simulink model "MHILSimTDFixpoint"  (R2021b)
settings: Solver=VariableStepAuto  StartTime=0.0  StopTime=10.0  RelTol=1e-3
values from neighbouring files (symbols this model uses):
  m = tddbl_model    [HILSimModel.m]
libraries: simulink x54
(part 1 of 2)
settings Model: Creator=berndorfer  LastModifiedBy=berndorfer

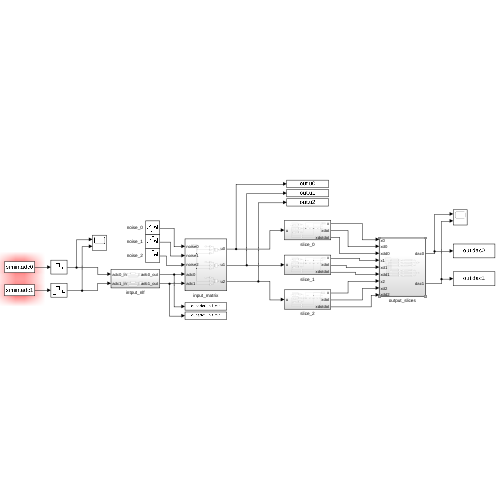
[thumbnail: Simulink's stored preview of the top-level diagram]
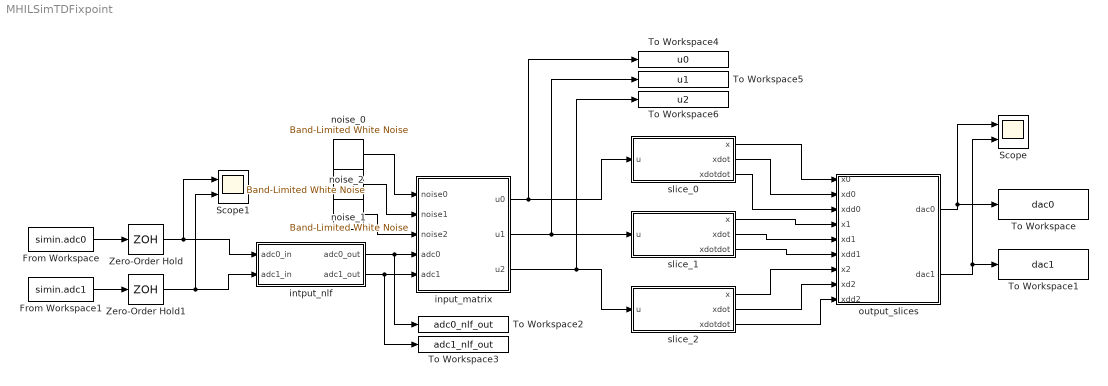
== system MHILSimTDFixpoint ==
  From Workspace : FromWorkspace  VariableName=simin.adc0
  From Workspace1 : FromWorkspace  VariableName=simin.adc1
  Scope : Scope  NumInputPorts=2
  Scope1 : Scope  NumInputPorts=2
  To Workspace : ToWorkspace  VariableName=dac0  SaveFormat=Timeseries  SampleTime=-1
  To Workspace1 : ToWorkspace  VariableName=dac1  SaveFormat=Timeseries  SampleTime=-1
  To Workspace2 : ToWorkspace  VariableName=adc0_nlf_out  SaveFormat=Timeseries  SampleTime=-1
  To Workspace3 : ToWorkspace  VariableName=adc1_nlf_out  SaveFormat=Timeseries  SampleTime=-1
  To Workspace4 : ToWorkspace  VariableName=u0  SaveFormat=Timeseries  SampleTime=-1
  To Workspace5 : ToWorkspace  VariableName=u1  SaveFormat=Timeseries  SampleTime=-1
  To Workspace6 : ToWorkspace  VariableName=u2  SaveFormat=Timeseries  SampleTime=-1
  Zero-Order Hold : ZeroOrderHold  SampleTime=m.t_s
  Zero-Order Hold1 : ZeroOrderHold  SampleTime=m.t_s
  input_matrix : Subsystem
  intput_nlf : Subsystem
  noise_0 : simulink/Sources/Band-Limited White Noise  Cov=[m.n0_power*m.t_s]  Ts=m.t_s  seed=[23341]
  noise_1 : simulink/Sources/Band-Limited White Noise  Cov=[m.n1_power*m.t_s]  Ts=m.t_s  seed=[23341]
  noise_2 : simulink/Sources/Band-Limited White Noise  Cov=[m.n2_power*m.t_s]  Ts=m.t_s  seed=[23341]
  output_slices : Subsystem
  slice_0 : Subsystem
  slice_1 : Subsystem
  slice_2 : Subsystem
  wires:
  slice_1/1(x) -> output_slices/4(x1)
  slice_1/2(xdot) -> output_slices/5(xd1)
  slice_0/2(xdot) -> output_slices/2(xd0)
  slice_0/1(x) -> output_slices/1(x0)
  slice_2/1(x) -> output_slices/7(x2)
  slice_2/2(xdot) -> output_slices/8(xd2)
  input_matrix/2(u1) -> To Workspace5/1, slice_1/1(u)
  input_matrix/1(u0) -> To Workspace4/1, slice_0/1(u)
  input_matrix/3(u2) -> To Workspace6/1, slice_2/1(u)
  intput_nlf/1(adc0_out) -> To Workspace2/1, input_matrix/4(adc0)
  intput_nlf/2(adc1_out) -> To Workspace3/1, input_matrix/5(adc1)
  output_slices/2(dac1) -> Scope/2, To Workspace1/1
  output_slices/1(dac0) -> Scope/1, To Workspace/1
  noise_0/1 -> input_matrix/1(noise0)
  noise_1/1 -> input_matrix/2(noise1)
  noise_2/1 -> input_matrix/3(noise2)
  From Workspace/1 -> Zero-Order Hold/1
  From Workspace1/1 -> Zero-Order Hold1/1
  Zero-Order Hold1/1 -> Scope1/2, intput_nlf/2(adc1_in)
  Zero-Order Hold/1 -> intput_nlf/1(adc0_in), Scope1/1
  slice_0/3(xdotdot) -> output_slices/3(xdd0)
  slice_1/3(xdotdot) -> output_slices/6(xdd1)
  slice_2/3(xdotdot) -> output_slices/9(xdd2)

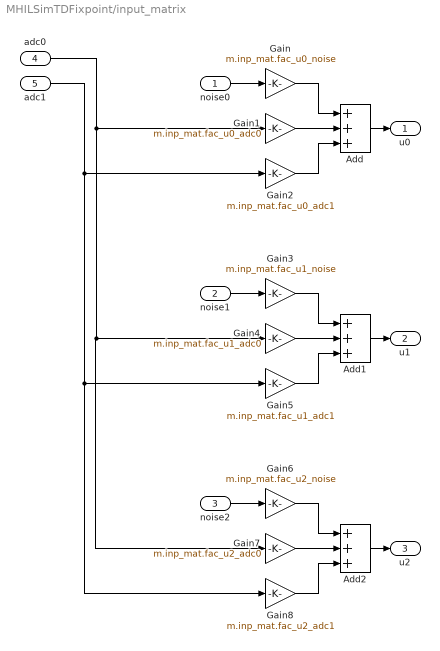
== system MHILSimTDFixpoint/input_matrix ==
  noise0 : Inport
  noise1 : Inport  Port=2
  noise2 : Inport  Port=3
  adc0 : Inport  Port=4
  adc1 : Inport  Port=5
  Add : Sum  Inputs=+++  OutDataTypeStr=m.datatype.slice
  Add1 : Sum  Inputs=+++  OutDataTypeStr=m.datatype.slice
  Add2 : Sum  Inputs=+++  OutDataTypeStr=m.datatype.slice
  Gain : Gain  Gain=m.inp_mat.fac_u0_noise  OutDataTypeStr=m.datatype.slice
  Gain1 : Gain  Gain=m.inp_mat.fac_u0_adc0  OutDataTypeStr=m.datatype.slice
  Gain2 : Gain  Gain=m.inp_mat.fac_u0_adc1  OutDataTypeStr=m.datatype.slice
  Gain3 : Gain  Gain=m.inp_mat.fac_u1_noise  OutDataTypeStr=m.datatype.slice
  Gain4 : Gain  Gain=m.inp_mat.fac_u1_adc0  OutDataTypeStr=m.datatype.slice
  Gain5 : Gain  Gain=m.inp_mat.fac_u1_adc1  OutDataTypeStr=m.datatype.slice
  Gain6 : Gain  Gain=m.inp_mat.fac_u2_noise  OutDataTypeStr=m.datatype.slice
  Gain7 : Gain  Gain=m.inp_mat.fac_u2_adc0  OutDataTypeStr=m.datatype.slice
  Gain8 : Gain  Gain=m.inp_mat.fac_u2_adc1  OutDataTypeStr=m.datatype.slice
  u0 : Outport
  u1 : Outport  Port=2
  u2 : Outport  Port=3
  wires:
  noise0/1 -> Gain/1
  Gain1/1 -> Add/2
  Gain/1 -> Add/1
  Gain2/1 -> Add/3
  adc0/1 -> Gain7/1, Gain4/1, Gain1/1
  adc1/1 -> Gain5/1, Gain8/1, Gain2/1
  Add/1 -> u0/1
  noise1/1 -> Gain3/1
  Gain4/1 -> Add1/2
  Gain5/1 -> Add1/3
  Add1/1 -> u1/1
  Gain3/1 -> Add1/1
  noise2/1 -> Gain6/1
  Gain7/1 -> Add2/2
  Gain8/1 -> Add2/3
  Add2/1 -> u2/1
  Gain6/1 -> Add2/1

== system MHILSimTDFixpoint/intput_nlf ==
  adc0_in : Inport
  adc1_in : Inport  Port=2
  Constant : Constant  Value=m.adc0_nlf.enabled
  Constant1 : Constant  Value=m.adc1_nlf.enabled
  Switch : Switch  Criteria=u2 ~= 0
  Switch1 : Switch  Criteria=u2 ~= 0
  adc0_nlf : Subsystem
  adc1_nlf : Subsystem
  adc0_out : Outport
  adc1_out : Outport  Port=2
  wires:
  adc1_nlf/1(f(x)) -> Switch1/1
  adc1_in/1 -> adc1_nlf/1(x), Switch1/3
  adc0_nlf/1(f(x)) -> Switch/1
  adc0_in/1 -> Switch/3, adc0_nlf/1(x)
  Constant/1 -> Switch/2
  Switch/1 -> adc0_out/1
  Constant1/1 -> Switch1/2
  Switch1/1 -> adc1_out/1

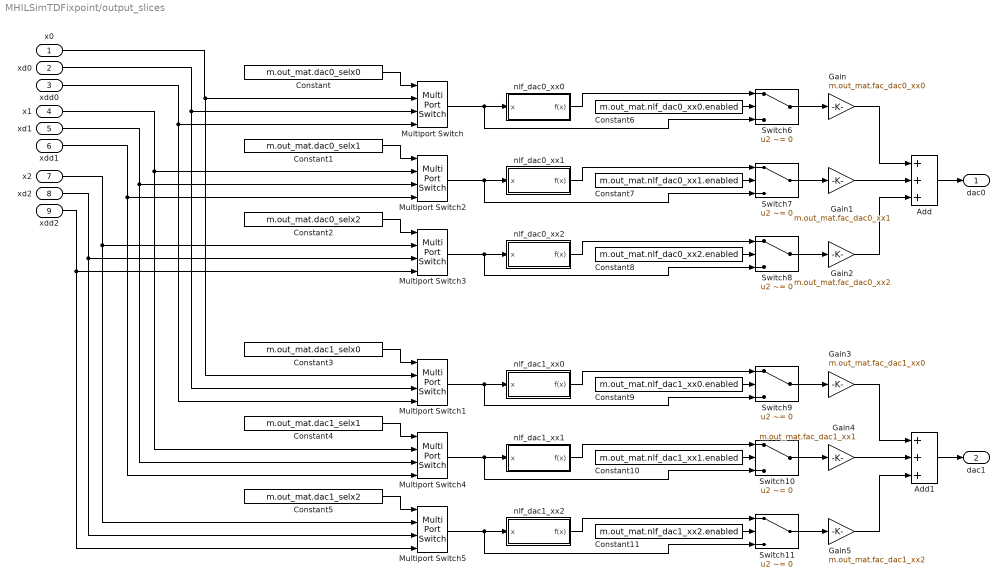
== system MHILSimTDFixpoint/output_slices ==
  x0 : Inport
  xd0 : Inport  Port=2
  xdd0 : Inport  Port=3
  x1 : Inport  Port=4
  xd1 : Inport  Port=5
  xdd1 : Inport  Port=6
  x2 : Inport  Port=7
  xd2 : Inport  Port=8
  xdd2 : Inport  Port=9
  Add : Sum  Inputs=+++  OutDataTypeStr=m.datatype.slice
  Add1 : Sum  Inputs=+++  OutDataTypeStr=m.datatype.slice
  Constant : Constant  Value=m.out_mat.dac0_selx0
  Constant1 : Constant  Value=m.out_mat.dac0_selx1
  Constant10 : Constant  Value=m.out_mat.nlf_dac1_xx1.enabled
  Constant11 : Constant  Value=m.out_mat.nlf_dac1_xx2.enabled
  Constant2 : Constant  Value=m.out_mat.dac0_selx2
  Constant3 : Constant  Value=m.out_mat.dac1_selx0
  Constant4 : Constant  Value=m.out_mat.dac1_selx1
  Constant5 : Constant  Value=m.out_mat.dac1_selx2
  Constant6 : Constant  Value=m.out_mat.nlf_dac0_xx0.enabled
  Constant7 : Constant  Value=m.out_mat.nlf_dac0_xx1.enabled
  Constant8 : Constant  Value=m.out_mat.nlf_dac0_xx2.enabled
  Constant9 : Constant  Value=m.out_mat.nlf_dac1_xx0.enabled
  Gain : Gain  Gain=m.out_mat.fac_dac0_xx0  OutDataTypeStr=m.datatype.slice
  Gain1 : Gain  Gain=m.out_mat.fac_dac0_xx1  OutDataTypeStr=m.datatype.slice
  Gain2 : Gain  Gain=m.out_mat.fac_dac0_xx2  OutDataTypeStr=m.datatype.slice
  Gain3 : Gain  Gain=m.out_mat.fac_dac1_xx0  OutDataTypeStr=m.datatype.slice
  Gain4 : Gain  Gain=m.out_mat.fac_dac1_xx1  OutDataTypeStr=m.datatype.slice
  Gain5 : Gain  Gain=m.out_mat.fac_dac1_xx2  OutDataTypeStr=m.datatype.slice
  Multiport Switch{,1..5} (6 alike) : MultiPortSwitch  DataPortOrder=Zero-based contiguous  zeroidx=on
  Switch{6..11} (6 alike) : Switch  Criteria=u2 ~= 0
  nlf_dac0_xx0 : Subsystem
  nlf_dac0_xx1 : Subsystem
  nlf_dac0_xx2 : Subsystem
  nlf_dac1_xx0 : Subsystem
  nlf_dac1_xx1 : Subsystem
  nlf_dac1_xx2 : Subsystem
  dac0 : Outport
  dac1 : Outport  Port=2
  wires:
  Gain1/1 -> Add/2
  Gain/1 -> Add/1
  Gain2/1 -> Add/3
  Add/1 -> dac0/1
  Gain4/1 -> Add1/2
  Gain3/1 -> Add1/1
  Gain5/1 -> Add1/3
  x0/1 -> Multiport Switch1/2, Multiport Switch/2
  xd0/1 -> Multiport Switch1/3, Multiport Switch/3
  Add1/1 -> dac1/1
  nlf_dac0_xx0/1(f(x)) -> Switch6/1
  Constant6/1 -> Switch6/2
  Switch6/1 -> Gain/1
  Multiport Switch/1 -> Switch6/3, nlf_dac0_xx0/1(x)
  nlf_dac0_xx1/1(f(x)) -> Switch7/1
  Multiport Switch2/1 -> Switch7/3, nlf_dac0_xx1/1(x)
  Constant7/1 -> Switch7/2
  nlf_dac0_xx2/1(f(x)) -> Switch8/1
  Multiport Switch3/1 -> Switch8/3, nlf_dac0_xx2/1(x)
  Constant8/1 -> Switch8/2
  Switch8/1 -> Gain2/1
  Switch7/1 -> Gain1/1
  nlf_dac1_xx0/1(f(x)) -> Switch9/1
  Multiport Switch5/1 -> Switch11/3, nlf_dac1_xx2/1(x)
  Switch9/1 -> Gain3/1
  Constant11/1 -> Switch11/2
  nlf_dac1_xx2/1(f(x)) -> Switch11/1
  Multiport Switch4/1 -> Switch10/3, nlf_dac1_xx1/1(x)
  nlf_dac1_xx1/1(f(x)) -> Switch10/1
  Constant10/1 -> Switch10/2
  Constant9/1 -> Switch9/2
  Multiport Switch1/1 -> Switch9/3, nlf_dac1_xx0/1(x)
  Switch10/1 -> Gain4/1
  Switch11/1 -> Gain5/1
  Constant/1 -> Multiport Switch/1
  xdd0/1 -> Multiport Switch1/4, Multiport Switch/4
  Constant3/1 -> Multiport Switch1/1
  x1/1 -> Multiport Switch4/2, Multiport Switch2/2
  Constant4/1 -> Multiport Switch4/1
  Constant5/1 -> Multiport Switch5/1
  Constant2/1 -> Multiport Switch3/1
  Constant1/1 -> Multiport Switch2/1
  xd1/1 -> Multiport Switch4/3, Multiport Switch2/3
  xdd1/1 -> Multiport Switch4/4, Multiport Switch2/4
  x2/1 -> Multiport Switch5/2, Multiport Switch3/2
  xd2/1 -> Multiport Switch5/3, Multiport Switch3/3
  xdd2/1 -> Multiport Switch5/4, Multiport Switch3/4

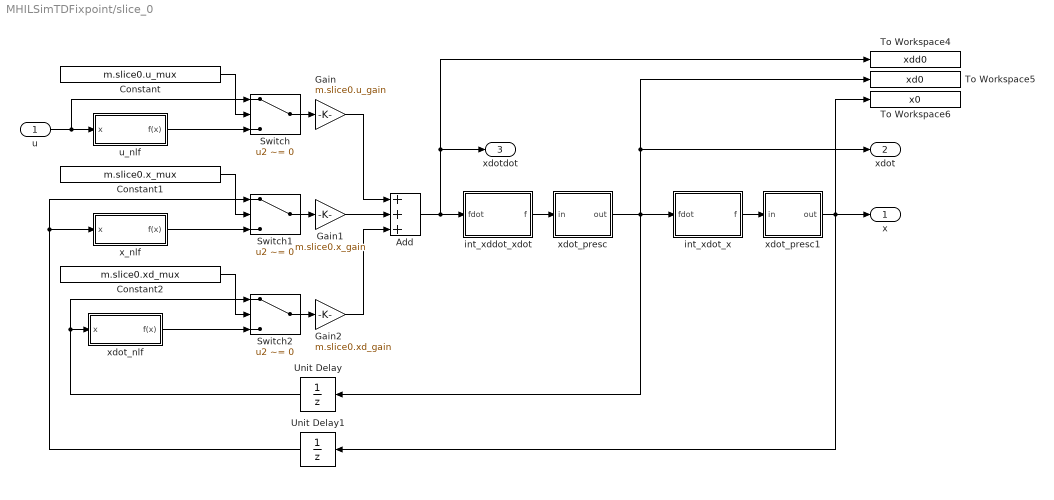
== system MHILSimTDFixpoint/slice_0 ==
  u : Inport
  Add : Sum  Inputs=+++  OutDataTypeStr=m.datatype.slice  SaturateOnIntegerOverflow=on
  Constant : Constant  Value=m.slice0.u_mux
  Constant1 : Constant  Value=m.slice0.x_mux
  Constant2 : Constant  Value=m.slice0.xd_mux
  Gain : Gain  Gain=m.slice0.u_gain  OutDataTypeStr=m.datatype.slice
  Gain1 : Gain  Gain=m.slice0.x_gain  OutDataTypeStr=m.datatype.slice
  Gain2 : Gain  Gain=m.slice0.xd_gain  OutDataTypeStr=m.datatype.slice
  Switch : Switch  Criteria=u2 ~= 0
  Switch1 : Switch  Criteria=u2 ~= 0
  Switch2 : Switch  Criteria=u2 ~= 0
  To Workspace4 : ToWorkspace  VariableName=xdd0  SaveFormat=Timeseries  SampleTime=-1
  To Workspace5 : ToWorkspace  VariableName=xd0  SaveFormat=Timeseries  SampleTime=-1
  To Workspace6 : ToWorkspace  VariableName=x0  SaveFormat=Timeseries  SampleTime=-1
  Unit Delay : UnitDelay  SampleTime=m.t_s  HasFrameUpgradeWarning=on
  Unit Delay1 : UnitDelay  SampleTime=m.t_s  HasFrameUpgradeWarning=on
  int_xddot_xdot : Subsystem
  int_xdot_x : Subsystem
  u_nlf : Subsystem
  x_nlf : Subsystem
  xdot_nlf : Subsystem
  xdot_presc : Subsystem
  xdot_presc1 : Subsystem
  x : Outport
  xdot : Outport  Port=2
  xdotdot : Outport  Port=3
  wires:
  Gain1/1 -> Add/2
  Gain2/1 -> Add/3
  Gain/1 -> Add/1
  u/1 -> Switch/1, u_nlf/1(x)
  Add/1 -> int_xddot_xdot/1(fdot), xdotdot/1, To Workspace4/1
  int_xddot_xdot/1(f) -> xdot_presc/1(in)
  int_xdot_x/1(f) -> xdot_presc1/1(in)
  xdot_presc/1(out) -> int_xdot_x/1(fdot), To Workspace5/1, xdot/1, Unit Delay/1
  Constant/1 -> Switch/2
  Switch/1 -> Gain/1
  u_nlf/1(f(x)) -> Switch/3
  Constant1/1 -> Switch1/2
  Switch1/1 -> Gain1/1
  x_nlf/1(f(x)) -> Switch1/3
  xdot_presc1/1(out) -> To Workspace6/1, x/1, Unit Delay1/1
  Constant2/1 -> Switch2/2
  Switch2/1 -> Gain2/1
  xdot_nlf/1(f(x)) -> Switch2/3
  Unit Delay/1 -> Switch2/1, xdot_nlf/1(x)
  Unit Delay1/1 -> x_nlf/1(x), Switch1/1

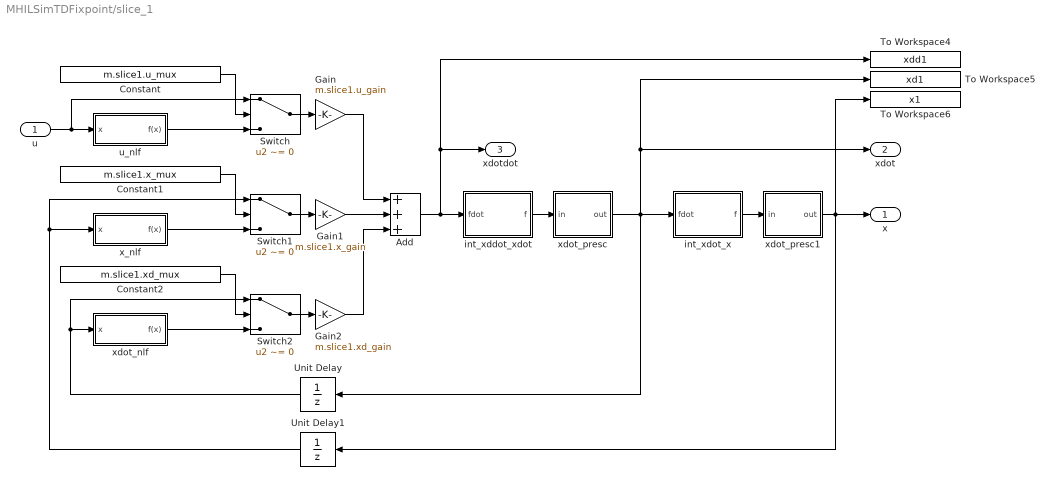
== system MHILSimTDFixpoint/slice_1 ==
  u : Inport
  Add : Sum  Inputs=+++  OutDataTypeStr=m.datatype.slice  SaturateOnIntegerOverflow=on
  Constant : Constant  Value=m.slice1.u_mux
  Constant1 : Constant  Value=m.slice1.x_mux
  Constant2 : Constant  Value=m.slice1.xd_mux
  Gain : Gain  Gain=m.slice1.u_gain  OutDataTypeStr=m.datatype.slice
  Gain1 : Gain  Gain=m.slice1.x_gain  OutDataTypeStr=m.datatype.slice
  Gain2 : Gain  Gain=m.slice1.xd_gain  OutDataTypeStr=m.datatype.slice
  Switch : Switch  Criteria=u2 ~= 0
  Switch1 : Switch  Criteria=u2 ~= 0
  Switch2 : Switch  Criteria=u2 ~= 0
  To Workspace4 : ToWorkspace  VariableName=xdd1  SaveFormat=Timeseries  SampleTime=-1
  To Workspace5 : ToWorkspace  VariableName=xd1  SaveFormat=Timeseries  SampleTime=-1
  To Workspace6 : ToWorkspace  VariableName=x1  SaveFormat=Timeseries  SampleTime=-1
  Unit Delay : UnitDelay  SampleTime=m.t_s  HasFrameUpgradeWarning=on
  Unit Delay1 : UnitDelay  SampleTime=m.t_s  HasFrameUpgradeWarning=on
  int_xddot_xdot : Subsystem
  int_xdot_x : Subsystem
  u_nlf : Subsystem
  x_nlf : Subsystem
  xdot_nlf : Subsystem
  xdot_presc : Subsystem
  xdot_presc1 : Subsystem
  x : Outport
  xdot : Outport  Port=2
  xdotdot : Outport  Port=3
  wires:
  Gain1/1 -> Add/2
  Gain2/1 -> Add/3
  Gain/1 -> Add/1
  u/1 -> Switch/1, u_nlf/1(x)
  Add/1 -> int_xddot_xdot/1(fdot), xdotdot/1, To Workspace4/1
  int_xddot_xdot/1(f) -> xdot_presc/1(in)
  int_xdot_x/1(f) -> xdot_presc1/1(in)
  xdot_presc/1(out) -> int_xdot_x/1(fdot), To Workspace5/1, xdot/1, Unit Delay/1
  Constant/1 -> Switch/2
  Switch/1 -> Gain/1
  u_nlf/1(f(x)) -> Switch/3
  Constant1/1 -> Switch1/2
  Switch1/1 -> Gain1/1
  x_nlf/1(f(x)) -> Switch1/3
  xdot_presc1/1(out) -> To Workspace6/1, x/1, Unit Delay1/1
  Constant2/1 -> Switch2/2
  Switch2/1 -> Gain2/1
  xdot_nlf/1(f(x)) -> Switch2/3
  Unit Delay/1 -> Switch2/1, xdot_nlf/1(x)
  Unit Delay1/1 -> Switch1/1, x_nlf/1(x)

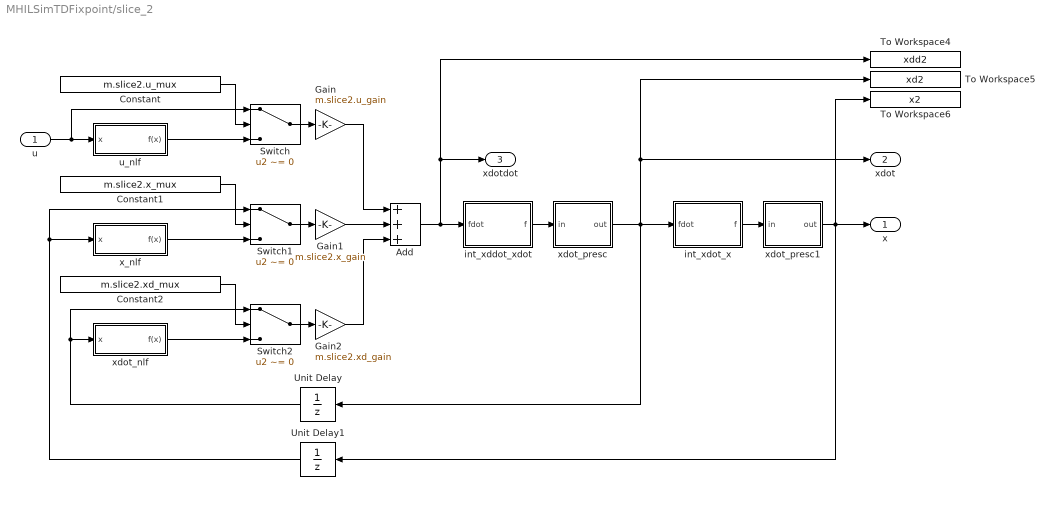
== system MHILSimTDFixpoint/slice_2 ==
  u : Inport
  Add : Sum  Inputs=+++  OutDataTypeStr=m.datatype.slice  SaturateOnIntegerOverflow=on
  Constant : Constant  Value=m.slice2.u_mux
  Constant1 : Constant  Value=m.slice2.x_mux
  Constant2 : Constant  Value=m.slice2.xd_mux
  Gain : Gain  Gain=m.slice2.u_gain  OutDataTypeStr=m.datatype.slice
  Gain1 : Gain  Gain=m.slice2.x_gain  OutDataTypeStr=m.datatype.slice
  Gain2 : Gain  Gain=m.slice2.xd_gain  OutDataTypeStr=m.datatype.slice
  Switch : Switch  Criteria=u2 ~= 0
  Switch1 : Switch  Criteria=u2 ~= 0
  Switch2 : Switch  Criteria=u2 ~= 0
  To Workspace4 : ToWorkspace  VariableName=xdd2  SaveFormat=Timeseries  SampleTime=-1
  To Workspace5 : ToWorkspace  VariableName=xd2  SaveFormat=Timeseries  SampleTime=-1
  To Workspace6 : ToWorkspace  VariableName=x2  SaveFormat=Timeseries  SampleTime=-1
  Unit Delay : UnitDelay  SampleTime=m.t_s  HasFrameUpgradeWarning=on
  Unit Delay1 : UnitDelay  SampleTime=m.t_s  HasFrameUpgradeWarning=on
  int_xddot_xdot : Subsystem
  int_xdot_x : Subsystem
  u_nlf : Subsystem
  x_nlf : Subsystem
  xdot_nlf : Subsystem
  xdot_presc : Subsystem
  xdot_presc1 : Subsystem
  x : Outport
  xdot : Outport  Port=2
  xdotdot : Outport  Port=3
  wires:
  Gain1/1 -> Add/2
  Gain2/1 -> Add/3
  Gain/1 -> Add/1
  u/1 -> Switch/1, u_nlf/1(x)
  int_xddot_xdot/1(f) -> xdot_presc/1(in)
  int_xdot_x/1(f) -> xdot_presc1/1(in)
  xdot_presc/1(out) -> To Workspace5/1, xdot/1, Unit Delay/1, int_xdot_x/1(fdot)
  Constant/1 -> Switch/2
  Switch/1 -> Gain/1
  u_nlf/1(f(x)) -> Switch/3
  Constant1/1 -> Switch1/2
  Switch1/1 -> Gain1/1
  x_nlf/1(f(x)) -> Switch1/3
  xdot_presc1/1(out) -> To Workspace6/1, x/1, Unit Delay1/1
  Constant2/1 -> Switch2/2
  Switch2/1 -> Gain2/1
  xdot_nlf/1(f(x)) -> Switch2/3
  Unit Delay/1 -> Switch2/1, xdot_nlf/1(x)
  Unit Delay1/1 -> Switch1/1, x_nlf/1(x)
  Add/1 -> xdotdot/1, To Workspace4/1, int_xddot_xdot/1(fdot)

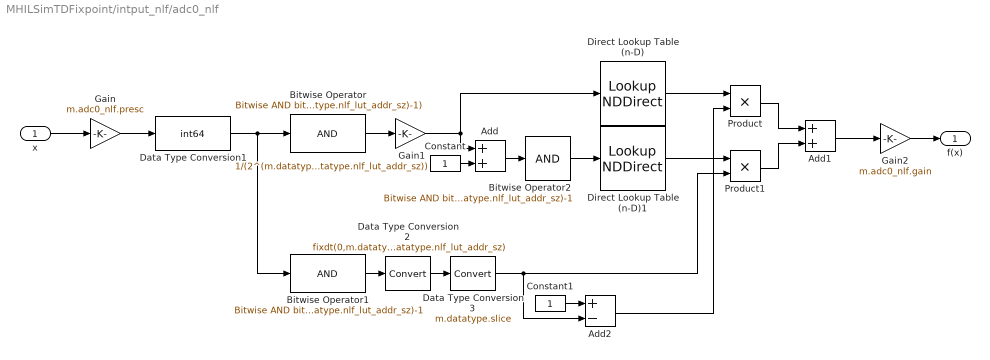
== system MHILSimTDFixpoint/intput_nlf/adc0_nlf ==
  x : Inport
  Add : Sum  OutDataTypeStr=uint64
  Add1 : Sum  OutDataTypeStr=m.datatype.slice
  Add2 : Sum  Inputs=+-  OutDataTypeStr=m.datatype.slice
  Bitwise Operator : simulink/Logic and Bit Operations/Bitwise Operator  logicop=AND  UseBitMask=on  BitMask=bitxor((bitsll(1,m.datatype.slice_sz)-1), bitsll(1,m.datatype.slice_sz - m.datatype.nlf_lut_addr_sz)-1)  BitMaskRealWorld=Stored Integer
  Bitwise Operator1 : simulink/Logic and Bit Operations/Bitwise Operator  logicop=AND  UseBitMask=on  BitMask=bitsll(1,m.datatype.slice_sz - m.datatype.nlf_lut_addr_sz)-1  BitMaskRealWorld=Stored Integer
  Bitwise Operator2 : simulink/Logic and Bit Operations/Bitwise Operator  logicop=AND  UseBitMask=on  BitMask=bitsll(1,m.datatype.nlf_lut_addr_sz)-1  BitMaskRealWorld=Stored Integer
  Constant : Constant  OutDataTypeStr=uint64
  Constant1 : Constant  OutDataTypeStr=m.datatype.const
  Data Type Conversion1 : DataTypeConversion  OutDataTypeStr=int64  ConvertRealWorld=Stored Integer (SI)
  Data Type Conversion2 : DataTypeConversion  OutDataTypeStr=fixdt(0,m.datatype.slice_sz - m.datatype.nlf_lut_addr_sz,m.datatype.slice_sz - m.datatype.nlf_lut_addr_sz)  ConvertRealWorld=Stored Integer (SI)
  Data Type Conversion3 : DataTypeConversion  OutDataTypeStr=m.datatype.slice
  Direct Lookup Table (n-D) : LookupNDDirect  NumberOfTableDimensions=1  Table=m.adc0_nlf.lut  TableDataTypeStr=m.datatype.nlf
  Direct Lookup Table (n-D)1 : LookupNDDirect  NumberOfTableDimensions=1  Table=m.adc0_nlf.lut  TableDataTypeStr=m.datatype.nlf
  Gain : Gain  Gain=m.adc0_nlf.presc  OutDataTypeStr=fixdt(1,m.datatype.slice_sz,m.datatype.slice_sz-1)
  Gain1 : Gain  Gain=1/(2^(m.datatype.slice_sz - m.datatype.nlf_lut_addr_sz))  OutDataTypeStr=uint64
  Gain2 : Gain  Gain=m.adc0_nlf.gain  OutDataTypeStr=m.datatype.slice
  Product : Product  OutDataTypeStr=m.datatype.slice
  Product1 : Product  OutDataTypeStr=m.datatype.slice
  f(x) : Outport
  wires:
  Direct Lookup Table (n-D)/1 -> Product/1
  Data Type Conversion2/1 -> Data Type Conversion3/1
  Product1/1 -> Add1/2
  Direct Lookup Table (n-D)1/1 -> Product1/1
  Bitwise Operator/1 -> Gain1/1
  Add2/1 -> Product/2
  Gain1/1 -> Add/1, Direct Lookup Table (n-D)/1
  Gain/1 -> Data Type Conversion1/1
  Data Type Conversion3/1 -> Product1/2, Add2/2
  Data Type Conversion1/1 -> Bitwise Operator1/1, Bitwise Operator/1
  Add1/1 -> Gain2/1
  Constant1/1 -> Add2/1
  Constant/1 -> Add/2
  Product/1 -> Add1/1
  Bitwise Operator1/1 -> Data Type Conversion2/1
  Add/1 -> Bitwise Operator2/1
  x/1 -> Gain/1
  Gain2/1 -> f(x)/1
  Bitwise Operator2/1 -> Direct Lookup Table (n-D)1/1

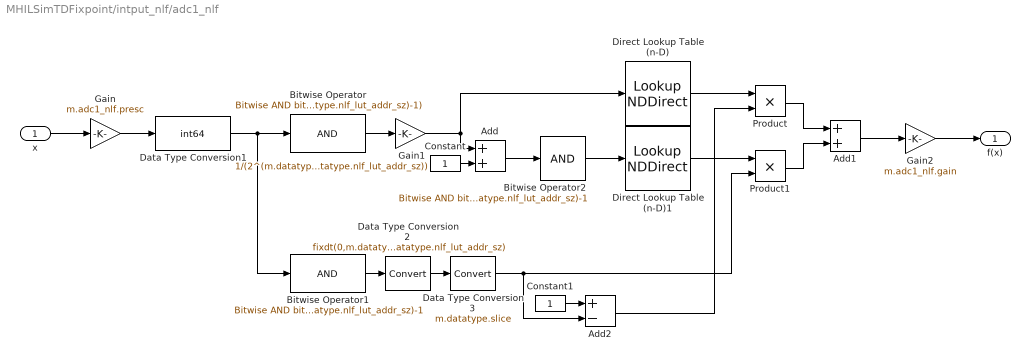
== system MHILSimTDFixpoint/intput_nlf/adc1_nlf ==
  x : Inport
  Add : Sum  OutDataTypeStr=uint64
  Add1 : Sum  OutDataTypeStr=m.datatype.slice
  Add2 : Sum  Inputs=+-  OutDataTypeStr=m.datatype.slice
  Bitwise Operator : simulink/Logic and Bit Operations/Bitwise Operator  logicop=AND  UseBitMask=on  BitMask=bitxor((bitsll(1,m.datatype.slice_sz)-1), bitsll(1,m.datatype.slice_sz - m.datatype.nlf_lut_addr_sz)-1)  BitMaskRealWorld=Stored Integer
  Bitwise Operator1 : simulink/Logic and Bit Operations/Bitwise Operator  logicop=AND  UseBitMask=on  BitMask=bitsll(1,m.datatype.slice_sz - m.datatype.nlf_lut_addr_sz)-1  BitMaskRealWorld=Stored Integer
  Bitwise Operator2 : simulink/Logic and Bit Operations/Bitwise Operator  logicop=AND  UseBitMask=on  BitMask=bitsll(1,m.datatype.nlf_lut_addr_sz)-1  BitMaskRealWorld=Stored Integer
  Constant : Constant  OutDataTypeStr=uint64
  Constant1 : Constant  OutDataTypeStr=m.datatype.const
  Data Type Conversion1 : DataTypeConversion  OutDataTypeStr=int64  ConvertRealWorld=Stored Integer (SI)
  Data Type Conversion2 : DataTypeConversion  OutDataTypeStr=fixdt(0,m.datatype.slice_sz - m.datatype.nlf_lut_addr_sz,m.datatype.slice_sz - m.datatype.nlf_lut_addr_sz)  ConvertRealWorld=Stored Integer (SI)
  Data Type Conversion3 : DataTypeConversion  OutDataTypeStr=m.datatype.slice
  Direct Lookup Table (n-D) : LookupNDDirect  NumberOfTableDimensions=1  Table=m.adc1_nlf.lut  TableDataTypeStr=m.datatype.nlf
  Direct Lookup Table (n-D)1 : LookupNDDirect  NumberOfTableDimensions=1  Table=m.adc1_nlf.lut  TableDataTypeStr=m.datatype.nlf
  Gain : Gain  Gain=m.adc1_nlf.presc  OutDataTypeStr=fixdt(1,m.datatype.slice_sz,m.datatype.slice_sz-1)
  Gain1 : Gain  Gain=1/(2^(m.datatype.slice_sz - m.datatype.nlf_lut_addr_sz))  OutDataTypeStr=uint64
  Gain2 : Gain  Gain=m.adc1_nlf.gain  OutDataTypeStr=m.datatype.slice
  Product : Product  OutDataTypeStr=m.datatype.slice
  Product1 : Product  OutDataTypeStr=m.datatype.slice
  f(x) : Outport
  wires:
  Direct Lookup Table (n-D)/1 -> Product/1
  Data Type Conversion2/1 -> Data Type Conversion3/1
  Product1/1 -> Add1/2
  Direct Lookup Table (n-D)1/1 -> Product1/1
  Bitwise Operator/1 -> Gain1/1
  Add2/1 -> Product/2
  Gain1/1 -> Add/1, Direct Lookup Table (n-D)/1
  Gain/1 -> Data Type Conversion1/1
  Data Type Conversion3/1 -> Product1/2, Add2/2
  Data Type Conversion1/1 -> Bitwise Operator1/1, Bitwise Operator/1
  Add1/1 -> Gain2/1
  Constant1/1 -> Add2/1
  Constant/1 -> Add/2
  Product/1 -> Add1/1
  Bitwise Operator1/1 -> Data Type Conversion2/1
  Add/1 -> Bitwise Operator2/1
  x/1 -> Gain/1
  Gain2/1 -> f(x)/1
  Bitwise Operator2/1 -> Direct Lookup Table (n-D)1/1

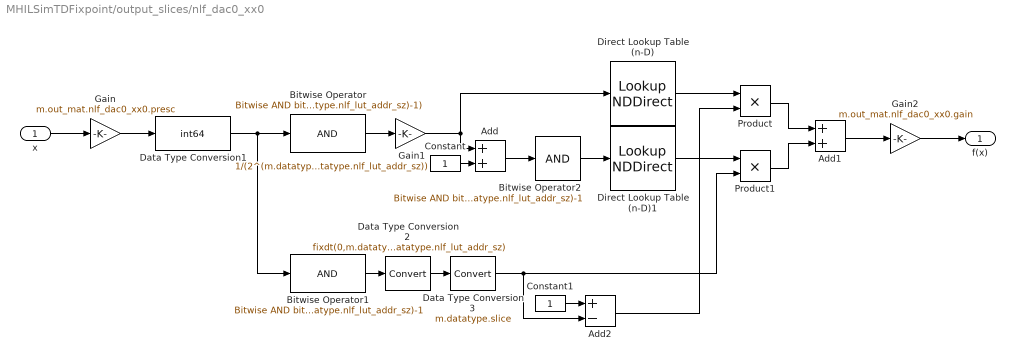
== system MHILSimTDFixpoint/output_slices/nlf_dac0_xx0 ==
  x : Inport
  Add : Sum  OutDataTypeStr=uint64
  Add1 : Sum  OutDataTypeStr=m.datatype.slice
  Add2 : Sum  Inputs=+-  OutDataTypeStr=m.datatype.slice
  Bitwise Operator : simulink/Logic and Bit Operations/Bitwise Operator  logicop=AND  UseBitMask=on  BitMask=bitxor((bitsll(1,m.datatype.slice_sz)-1), bitsll(1,m.datatype.slice_sz - m.datatype.nlf_lut_addr_sz)-1)  BitMaskRealWorld=Stored Integer
  Bitwise Operator1 : simulink/Logic and Bit Operations/Bitwise Operator  logicop=AND  UseBitMask=on  BitMask=bitsll(1,m.datatype.slice_sz - m.datatype.nlf_lut_addr_sz)-1  BitMaskRealWorld=Stored Integer
  Bitwise Operator2 : simulink/Logic and Bit Operations/Bitwise Operator  logicop=AND  UseBitMask=on  BitMask=bitsll(1,m.datatype.nlf_lut_addr_sz)-1  BitMaskRealWorld=Stored Integer
  Constant : Constant  OutDataTypeStr=uint64
  Constant1 : Constant  OutDataTypeStr=m.datatype.const
  Data Type Conversion1 : DataTypeConversion  OutDataTypeStr=int64  ConvertRealWorld=Stored Integer (SI)
  Data Type Conversion2 : DataTypeConversion  OutDataTypeStr=fixdt(0,m.datatype.slice_sz - m.datatype.nlf_lut_addr_sz,m.datatype.slice_sz - m.datatype.nlf_lut_addr_sz)  ConvertRealWorld=Stored Integer (SI)
  Data Type Conversion3 : DataTypeConversion  OutDataTypeStr=m.datatype.slice
  Direct Lookup Table (n-D) : LookupNDDirect  NumberOfTableDimensions=1  Table=m.out_mat.nlf_dac0_xx0.lut  TableDataTypeStr=m.datatype.nlf
  Direct Lookup Table (n-D)1 : LookupNDDirect  NumberOfTableDimensions=1  Table=m.out_mat.nlf_dac0_xx0.lut  TableDataTypeStr=m.datatype.nlf
  Gain : Gain  Gain=m.out_mat.nlf_dac0_xx0.presc  OutDataTypeStr=fixdt(1,m.datatype.slice_sz,m.datatype.slice_sz-1)
  Gain1 : Gain  Gain=1/(2^(m.datatype.slice_sz - m.datatype.nlf_lut_addr_sz))  OutDataTypeStr=uint64
  Gain2 : Gain  Gain=m.out_mat.nlf_dac0_xx0.gain  OutDataTypeStr=m.datatype.slice
  Product : Product  OutDataTypeStr=m.datatype.slice
  Product1 : Product  OutDataTypeStr=m.datatype.slice
  f(x) : Outport
  wires:
  Direct Lookup Table (n-D)/1 -> Product/1
  Data Type Conversion2/1 -> Data Type Conversion3/1
  Product1/1 -> Add1/2
  Direct Lookup Table (n-D)1/1 -> Product1/1
  Bitwise Operator/1 -> Gain1/1
  Add2/1 -> Product/2
  Gain1/1 -> Add/1, Direct Lookup Table (n-D)/1
  Gain/1 -> Data Type Conversion1/1
  Data Type Conversion3/1 -> Product1/2, Add2/2
  Data Type Conversion1/1 -> Bitwise Operator1/1, Bitwise Operator/1
  Add1/1 -> Gain2/1
  Constant1/1 -> Add2/1
  Constant/1 -> Add/2
  Product/1 -> Add1/1
  Bitwise Operator1/1 -> Data Type Conversion2/1
  Add/1 -> Bitwise Operator2/1
  x/1 -> Gain/1
  Gain2/1 -> f(x)/1
  Bitwise Operator2/1 -> Direct Lookup Table (n-D)1/1

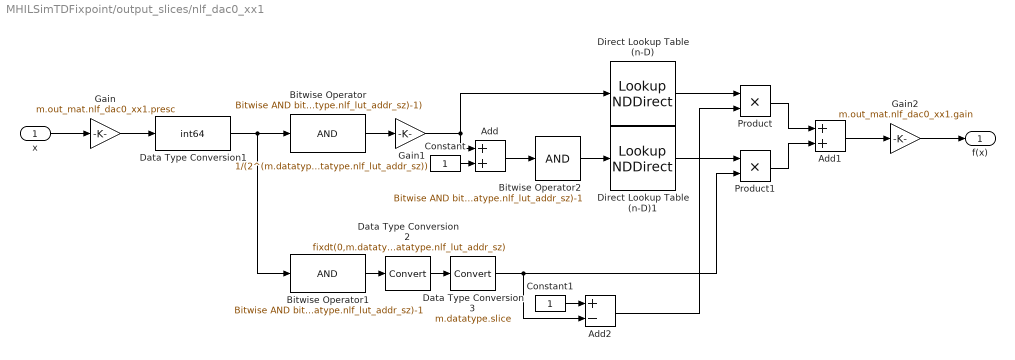
== system MHILSimTDFixpoint/output_slices/nlf_dac0_xx1 ==
  x : Inport
  Add : Sum  OutDataTypeStr=uint64
  Add1 : Sum  OutDataTypeStr=m.datatype.slice
  Add2 : Sum  Inputs=+-  OutDataTypeStr=m.datatype.slice
  Bitwise Operator : simulink/Logic and Bit Operations/Bitwise Operator  logicop=AND  UseBitMask=on  BitMask=bitxor((bitsll(1,m.datatype.slice_sz)-1), bitsll(1,m.datatype.slice_sz - m.datatype.nlf_lut_addr_sz)-1)  BitMaskRealWorld=Stored Integer
  Bitwise Operator1 : simulink/Logic and Bit Operations/Bitwise Operator  logicop=AND  UseBitMask=on  BitMask=bitsll(1,m.datatype.slice_sz - m.datatype.nlf_lut_addr_sz)-1  BitMaskRealWorld=Stored Integer
  Bitwise Operator2 : simulink/Logic and Bit Operations/Bitwise Operator  logicop=AND  UseBitMask=on  BitMask=bitsll(1,m.datatype.nlf_lut_addr_sz)-1  BitMaskRealWorld=Stored Integer
  Constant : Constant  OutDataTypeStr=uint64
  Constant1 : Constant  OutDataTypeStr=m.datatype.const
  Data Type Conversion1 : DataTypeConversion  OutDataTypeStr=int64  ConvertRealWorld=Stored Integer (SI)
  Data Type Conversion2 : DataTypeConversion  OutDataTypeStr=fixdt(0,m.datatype.slice_sz - m.datatype.nlf_lut_addr_sz,m.datatype.slice_sz - m.datatype.nlf_lut_addr_sz)  ConvertRealWorld=Stored Integer (SI)
  Data Type Conversion3 : DataTypeConversion  OutDataTypeStr=m.datatype.slice
  Direct Lookup Table (n-D) : LookupNDDirect  NumberOfTableDimensions=1  Table=m.out_mat.nlf_dac0_xx1.lut  TableDataTypeStr=m.datatype.nlf
  Direct Lookup Table (n-D)1 : LookupNDDirect  NumberOfTableDimensions=1  Table=m.out_mat.nlf_dac0_xx1.lut  TableDataTypeStr=m.datatype.nlf
  Gain : Gain  Gain=m.out_mat.nlf_dac0_xx1.presc  OutDataTypeStr=fixdt(1,m.datatype.slice_sz,m.datatype.slice_sz-1)
  Gain1 : Gain  Gain=1/(2^(m.datatype.slice_sz - m.datatype.nlf_lut_addr_sz))  OutDataTypeStr=uint64
  Gain2 : Gain  Gain=m.out_mat.nlf_dac0_xx1.gain  OutDataTypeStr=m.datatype.slice
  Product : Product  OutDataTypeStr=m.datatype.slice
  Product1 : Product  OutDataTypeStr=m.datatype.slice
  f(x) : Outport
  wires:
  Direct Lookup Table (n-D)/1 -> Product/1
  Data Type Conversion2/1 -> Data Type Conversion3/1
  Product1/1 -> Add1/2
  Direct Lookup Table (n-D)1/1 -> Product1/1
  Bitwise Operator/1 -> Gain1/1
  Add2/1 -> Product/2
  Gain1/1 -> Add/1, Direct Lookup Table (n-D)/1
  Gain/1 -> Data Type Conversion1/1
  Data Type Conversion3/1 -> Product1/2, Add2/2
  Data Type Conversion1/1 -> Bitwise Operator1/1, Bitwise Operator/1
  Add1/1 -> Gain2/1
  Constant1/1 -> Add2/1
  Constant/1 -> Add/2
  Product/1 -> Add1/1
  Bitwise Operator1/1 -> Data Type Conversion2/1
  Add/1 -> Bitwise Operator2/1
  x/1 -> Gain/1
  Gain2/1 -> f(x)/1
  Bitwise Operator2/1 -> Direct Lookup Table (n-D)1/1

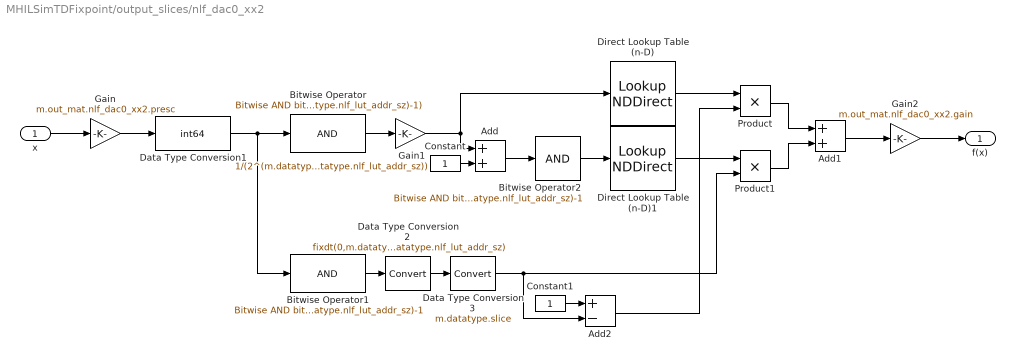
== system MHILSimTDFixpoint/output_slices/nlf_dac0_xx2 ==
  x : Inport
  Add : Sum  OutDataTypeStr=uint64
  Add1 : Sum  OutDataTypeStr=m.datatype.slice
  Add2 : Sum  Inputs=+-  OutDataTypeStr=m.datatype.slice
  Bitwise Operator : simulink/Logic and Bit Operations/Bitwise Operator  logicop=AND  UseBitMask=on  BitMask=bitxor((bitsll(1,m.datatype.slice_sz)-1), bitsll(1,m.datatype.slice_sz - m.datatype.nlf_lut_addr_sz)-1)  BitMaskRealWorld=Stored Integer
  Bitwise Operator1 : simulink/Logic and Bit Operations/Bitwise Operator  logicop=AND  UseBitMask=on  BitMask=bitsll(1,m.datatype.slice_sz - m.datatype.nlf_lut_addr_sz)-1  BitMaskRealWorld=Stored Integer
  Bitwise Operator2 : simulink/Logic and Bit Operations/Bitwise Operator  logicop=AND  UseBitMask=on  BitMask=bitsll(1,m.datatype.nlf_lut_addr_sz)-1  BitMaskRealWorld=Stored Integer
  Constant : Constant  OutDataTypeStr=uint64
  Constant1 : Constant  OutDataTypeStr=m.datatype.const
  Data Type Conversion1 : DataTypeConversion  OutDataTypeStr=int64  ConvertRealWorld=Stored Integer (SI)
  Data Type Conversion2 : DataTypeConversion  OutDataTypeStr=fixdt(0,m.datatype.slice_sz - m.datatype.nlf_lut_addr_sz,m.datatype.slice_sz - m.datatype.nlf_lut_addr_sz)  ConvertRealWorld=Stored Integer (SI)
  Data Type Conversion3 : DataTypeConversion  OutDataTypeStr=m.datatype.slice
  Direct Lookup Table (n-D) : LookupNDDirect  NumberOfTableDimensions=1  Table=m.out_mat.nlf_dac0_xx2.lut  TableDataTypeStr=m.datatype.nlf
  Direct Lookup Table (n-D)1 : LookupNDDirect  NumberOfTableDimensions=1  Table=m.out_mat.nlf_dac0_xx2.lut  TableDataTypeStr=m.datatype.nlf
  Gain : Gain  Gain=m.out_mat.nlf_dac0_xx2.presc  OutDataTypeStr=fixdt(1,m.datatype.slice_sz,m.datatype.slice_sz-1)
  Gain1 : Gain  Gain=1/(2^(m.datatype.slice_sz - m.datatype.nlf_lut_addr_sz))  OutDataTypeStr=uint64
  Gain2 : Gain  Gain=m.out_mat.nlf_dac0_xx2.gain  OutDataTypeStr=m.datatype.slice
  Product : Product  OutDataTypeStr=m.datatype.slice
  Product1 : Product  OutDataTypeStr=m.datatype.slice
  f(x) : Outport
  wires:
  Direct Lookup Table (n-D)/1 -> Product/1
  Data Type Conversion2/1 -> Data Type Conversion3/1
  Product1/1 -> Add1/2
  Direct Lookup Table (n-D)1/1 -> Product1/1
  Bitwise Operator/1 -> Gain1/1
  Add2/1 -> Product/2
  Gain1/1 -> Add/1, Direct Lookup Table (n-D)/1
  Gain/1 -> Data Type Conversion1/1
  Data Type Conversion3/1 -> Product1/2, Add2/2
  Data Type Conversion1/1 -> Bitwise Operator1/1, Bitwise Operator/1
  Add1/1 -> Gain2/1
  Constant1/1 -> Add2/1
  Constant/1 -> Add/2
  Product/1 -> Add1/1
  Bitwise Operator1/1 -> Data Type Conversion2/1
  Add/1 -> Bitwise Operator2/1
  x/1 -> Gain/1
  Gain2/1 -> f(x)/1
  Bitwise Operator2/1 -> Direct Lookup Table (n-D)1/1

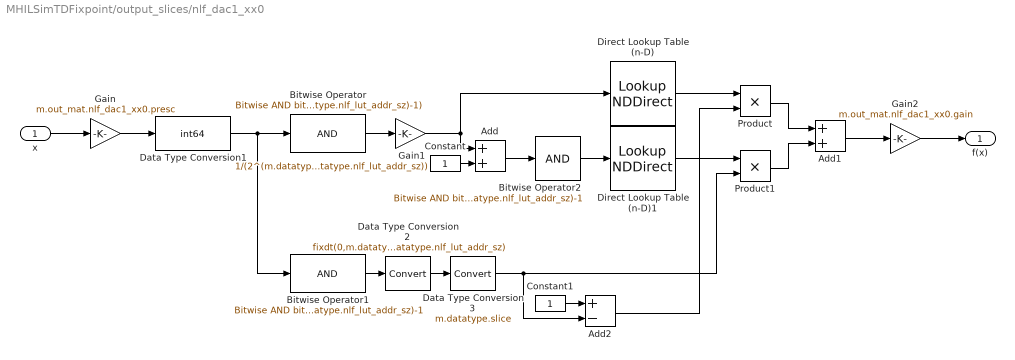
== system MHILSimTDFixpoint/output_slices/nlf_dac1_xx0 ==
  x : Inport
  Add : Sum  OutDataTypeStr=uint64
  Add1 : Sum  OutDataTypeStr=m.datatype.slice
  Add2 : Sum  Inputs=+-  OutDataTypeStr=m.datatype.slice
  Bitwise Operator : simulink/Logic and Bit Operations/Bitwise Operator  logicop=AND  UseBitMask=on  BitMask=bitxor((bitsll(1,m.datatype.slice_sz)-1), bitsll(1,m.datatype.slice_sz - m.datatype.nlf_lut_addr_sz)-1)  BitMaskRealWorld=Stored Integer
  Bitwise Operator1 : simulink/Logic and Bit Operations/Bitwise Operator  logicop=AND  UseBitMask=on  BitMask=bitsll(1,m.datatype.slice_sz - m.datatype.nlf_lut_addr_sz)-1  BitMaskRealWorld=Stored Integer
  Bitwise Operator2 : simulink/Logic and Bit Operations/Bitwise Operator  logicop=AND  UseBitMask=on  BitMask=bitsll(1,m.datatype.nlf_lut_addr_sz)-1  BitMaskRealWorld=Stored Integer
  Constant : Constant  OutDataTypeStr=uint64
  Constant1 : Constant  OutDataTypeStr=m.datatype.const
  Data Type Conversion1 : DataTypeConversion  OutDataTypeStr=int64  ConvertRealWorld=Stored Integer (SI)
  Data Type Conversion2 : DataTypeConversion  OutDataTypeStr=fixdt(0,m.datatype.slice_sz - m.datatype.nlf_lut_addr_sz,m.datatype.slice_sz - m.datatype.nlf_lut_addr_sz)  ConvertRealWorld=Stored Integer (SI)
  Data Type Conversion3 : DataTypeConversion  OutDataTypeStr=m.datatype.slice
  Direct Lookup Table (n-D) : LookupNDDirect  NumberOfTableDimensions=1  Table=m.out_mat.nlf_dac1_xx0.lut  TableDataTypeStr=m.datatype.nlf
  Direct Lookup Table (n-D)1 : LookupNDDirect  NumberOfTableDimensions=1  Table=m.out_mat.nlf_dac1_xx0.lut  TableDataTypeStr=m.datatype.nlf
  Gain : Gain  Gain=m.out_mat.nlf_dac1_xx0.presc  OutDataTypeStr=fixdt(1,m.datatype.slice_sz,m.datatype.slice_sz-1)
  Gain1 : Gain  Gain=1/(2^(m.datatype.slice_sz - m.datatype.nlf_lut_addr_sz))  OutDataTypeStr=uint64
  Gain2 : Gain  Gain=m.out_mat.nlf_dac1_xx0.gain  OutDataTypeStr=m.datatype.slice
  Product : Product  OutDataTypeStr=m.datatype.slice
  Product1 : Product  OutDataTypeStr=m.datatype.slice
  f(x) : Outport
  wires:
  Direct Lookup Table (n-D)/1 -> Product/1
  Data Type Conversion2/1 -> Data Type Conversion3/1
  Product1/1 -> Add1/2
  Direct Lookup Table (n-D)1/1 -> Product1/1
  Bitwise Operator/1 -> Gain1/1
  Add2/1 -> Product/2
  Gain1/1 -> Add/1, Direct Lookup Table (n-D)/1
  Gain/1 -> Data Type Conversion1/1
  Data Type Conversion3/1 -> Product1/2, Add2/2
  Data Type Conversion1/1 -> Bitwise Operator1/1, Bitwise Operator/1
  Add1/1 -> Gain2/1
  Constant1/1 -> Add2/1
  Constant/1 -> Add/2
  Product/1 -> Add1/1
  Bitwise Operator1/1 -> Data Type Conversion2/1
  Add/1 -> Bitwise Operator2/1
  x/1 -> Gain/1
  Gain2/1 -> f(x)/1
  Bitwise Operator2/1 -> Direct Lookup Table (n-D)1/1

== system MHILSimTDFixpoint/output_slices/nlf_dac1_xx1 ==
  x : Inport
  Add : Sum  OutDataTypeStr=uint64
  Add1 : Sum  OutDataTypeStr=m.datatype.slice
  Add2 : Sum  Inputs=+-  OutDataTypeStr=m.datatype.slice
  Bitwise Operator : simulink/Logic and Bit Operations/Bitwise Operator  logicop=AND  UseBitMask=on  BitMask=bitxor((bitsll(1,m.datatype.slice_sz)-1), bitsll(1,m.datatype.slice_sz - m.datatype.nlf_lut_addr_sz)-1)  BitMaskRealWorld=Stored Integer
  Bitwise Operator1 : simulink/Logic and Bit Operations/Bitwise Operator  logicop=AND  UseBitMask=on  BitMask=bitsll(1,m.datatype.slice_sz - m.datatype.nlf_lut_addr_sz)-1  BitMaskRealWorld=Stored Integer
  Bitwise Operator2 : simulink/Logic and Bit Operations/Bitwise Operator  logicop=AND  UseBitMask=on  BitMask=bitsll(1,m.datatype.nlf_lut_addr_sz)-1  BitMaskRealWorld=Stored Integer
  Constant : Constant  OutDataTypeStr=uint64
  Constant1 : Constant  OutDataTypeStr=m.datatype.const
  Data Type Conversion1 : DataTypeConversion  OutDataTypeStr=int64  ConvertRealWorld=Stored Integer (SI)
  Data Type Conversion2 : DataTypeConversion  OutDataTypeStr=fixdt(0,m.datatype.slice_sz - m.datatype.nlf_lut_addr_sz,m.datatype.slice_sz - m.datatype.nlf_lut_addr_sz)  ConvertRealWorld=Stored Integer (SI)
  Data Type Conversion3 : DataTypeConversion  OutDataTypeStr=m.datatype.slice
  Direct Lookup Table (n-D) : LookupNDDirect  NumberOfTableDimensions=1  Table=m.out_mat.nlf_dac1_xx1.lut  TableDataTypeStr=m.datatype.nlf
  Direct Lookup Table (n-D)1 : LookupNDDirect  NumberOfTableDimensions=1  Table=m.out_mat.nlf_dac1_xx1.lut  TableDataTypeStr=m.datatype.nlf
  Gain : Gain  Gain=m.out_mat.nlf_dac1_xx1.presc  OutDataTypeStr=fixdt(1,m.datatype.slice_sz,m.datatype.slice_sz-1)
  Gain1 : Gain  Gain=1/(2^(m.datatype.slice_sz - m.datatype.nlf_lut_addr_sz))  OutDataTypeStr=uint64
  Gain2 : Gain  Gain=m.out_mat.nlf_dac1_xx1.gain  OutDataTypeStr=m.datatype.slice
  Product : Product  OutDataTypeStr=m.datatype.slice
  Product1 : Product  OutDataTypeStr=m.datatype.slice
  f(x) : Outport
  wires:
  Direct Lookup Table (n-D)/1 -> Product/1
  Data Type Conversion2/1 -> Data Type Conversion3/1
  Product1/1 -> Add1/2
  Direct Lookup Table (n-D)1/1 -> Product1/1
  Bitwise Operator/1 -> Gain1/1
  Add2/1 -> Product/2
  Gain1/1 -> Add/1, Direct Lookup Table (n-D)/1
  Gain/1 -> Data Type Conversion1/1
  Data Type Conversion3/1 -> Product1/2, Add2/2
  Data Type Conversion1/1 -> Bitwise Operator1/1, Bitwise Operator/1
  Add1/1 -> Gain2/1
  Constant1/1 -> Add2/1
  Constant/1 -> Add/2
  Product/1 -> Add1/1
  Bitwise Operator1/1 -> Data Type Conversion2/1
  Add/1 -> Bitwise Operator2/1
  x/1 -> Gain/1
  Gain2/1 -> f(x)/1
  Bitwise Operator2/1 -> Direct Lookup Table (n-D)1/1

== system MHILSimTDFixpoint/output_slices/nlf_dac1_xx2 ==
  x : Inport
  Add : Sum  OutDataTypeStr=uint64
  Add1 : Sum  OutDataTypeStr=m.datatype.slice
  Add2 : Sum  Inputs=+-  OutDataTypeStr=m.datatype.slice
  Bitwise Operator : simulink/Logic and Bit Operations/Bitwise Operator  logicop=AND  UseBitMask=on  BitMask=bitxor((bitsll(1,m.datatype.slice_sz)-1), bitsll(1,m.datatype.slice_sz - m.datatype.nlf_lut_addr_sz)-1)  BitMaskRealWorld=Stored Integer
  Bitwise Operator1 : simulink/Logic and Bit Operations/Bitwise Operator  logicop=AND  UseBitMask=on  BitMask=bitsll(1,m.datatype.slice_sz - m.datatype.nlf_lut_addr_sz)-1  BitMaskRealWorld=Stored Integer
  Bitwise Operator2 : simulink/Logic and Bit Operations/Bitwise Operator  logicop=AND  UseBitMask=on  BitMask=bitsll(1,m.datatype.nlf_lut_addr_sz)-1  BitMaskRealWorld=Stored Integer
  Constant : Constant  OutDataTypeStr=uint64
  Constant1 : Constant  OutDataTypeStr=m.datatype.const
  Data Type Conversion1 : DataTypeConversion  OutDataTypeStr=int64  ConvertRealWorld=Stored Integer (SI)
  Data Type Conversion2 : DataTypeConversion  OutDataTypeStr=fixdt(0,m.datatype.slice_sz - m.datatype.nlf_lut_addr_sz,m.datatype.slice_sz - m.datatype.nlf_lut_addr_sz)  ConvertRealWorld=Stored Integer (SI)
  Data Type Conversion3 : DataTypeConversion  OutDataTypeStr=m.datatype.slice
  Direct Lookup Table (n-D) : LookupNDDirect  NumberOfTableDimensions=1  Table=m.out_mat.nlf_dac1_xx2.lut  TableDataTypeStr=m.datatype.nlf
  Direct Lookup Table (n-D)1 : LookupNDDirect  NumberOfTableDimensions=1  Table=m.out_mat.nlf_dac1_xx2.lut  TableDataTypeStr=m.datatype.nlf
  Gain : Gain  Gain=m.out_mat.nlf_dac1_xx2.presc  OutDataTypeStr=fixdt(1,m.datatype.slice_sz,m.datatype.slice_sz-1)
  Gain1 : Gain  Gain=1/(2^(m.datatype.slice_sz - m.datatype.nlf_lut_addr_sz))  OutDataTypeStr=uint64
  Gain2 : Gain  Gain=m.out_mat.nlf_dac1_xx2.gain  OutDataTypeStr=m.datatype.slice
  Product : Product  OutDataTypeStr=m.datatype.slice
  Product1 : Product  OutDataTypeStr=m.datatype.slice
  f(x) : Outport
  wires:
  Direct Lookup Table (n-D)/1 -> Product/1
  Data Type Conversion2/1 -> Data Type Conversion3/1
  Product1/1 -> Add1/2
  Direct Lookup Table (n-D)1/1 -> Product1/1
  Bitwise Operator/1 -> Gain1/1
  Add2/1 -> Product/2
  Gain1/1 -> Add/1, Direct Lookup Table (n-D)/1
  Gain/1 -> Data Type Conversion1/1
  Data Type Conversion3/1 -> Product1/2, Add2/2
  Data Type Conversion1/1 -> Bitwise Operator1/1, Bitwise Operator/1
  Add1/1 -> Gain2/1
  Constant1/1 -> Add2/1
  Constant/1 -> Add/2
  Product/1 -> Add1/1
  Bitwise Operator1/1 -> Data Type Conversion2/1
  Add/1 -> Bitwise Operator2/1
  x/1 -> Gain/1
  Gain2/1 -> f(x)/1
  Bitwise Operator2/1 -> Direct Lookup Table (n-D)1/1

== system MHILSimTDFixpoint/slice_0/int_xddot_xdot ==
  fdot : Inport
  Add : Sum  OutDataTypeStr=m.datatype.accum
  Add1 : Sum  Inputs=+-  OutDataTypeStr=m.datatype.slice
  Add2 : Sum  OutDataTypeStr=m.datatype.slice
  Unit Delay : UnitDelay  SampleTime=m.t_s  HasFrameUpgradeWarning=on
  Unit Delay1 : UnitDelay  SampleTime=m.t_s  HasFrameUpgradeWarning=on
  fp_prepend_zeros : DataTypeConversion  OutDataTypeStr=fixdt(1,m.datatype.slice_sz+m.int_scale_bits,m.datatype.slice_bin)
  fp_repr_shift_prescale : Gain  Gain=1/(2^m.int_scale_bits)  OutDataTypeStr=m.datatype.accum
  half : Gain  Gain=1/2  OutDataTypeStr=m.datatype.slice
  int_presc : Gain  Gain=m.int_dt_residual  OutDataTypeStr=m.datatype.slice
  f : Outport
  wires:
  int_presc/1 -> fp_prepend_zeros/1
  fp_repr_shift_prescale/1 -> Add/1
  Add/1 -> f/1, Unit Delay/1
  fp_prepend_zeros/1 -> fp_repr_shift_prescale/1
  Unit Delay/1 -> Add/2
  fdot/1 -> half/1, Add2/1
  Add1/1 -> int_presc/1
  Add2/1 -> Add1/1
  half/1 -> Add2/2, Unit Delay1/1
  Unit Delay1/1 -> Add1/2

== system MHILSimTDFixpoint/slice_0/int_xdot_x ==
  fdot : Inport
  Add : Sum  OutDataTypeStr=m.datatype.accum
  Add1 : Sum  OutDataTypeStr=m.datatype.slice
  Unit Delay : UnitDelay  SampleTime=m.t_s  HasFrameUpgradeWarning=on
  Unit Delay1 : UnitDelay  SampleTime=m.t_s  HasFrameUpgradeWarning=on
  fp_prepend_zeros : DataTypeConversion  OutDataTypeStr=fixdt(1,m.datatype.slice_sz+m.int_scale_bits,m.datatype.slice_bin)
  fp_repr_shift_prescale : Gain  Gain=1/(2^m.int_scale_bits)  OutDataTypeStr=m.datatype.accum
  half : Gain  Gain=1/2  OutDataTypeStr=m.datatype.slice
  int_presc : Gain  Gain=m.int_dt_residual  OutDataTypeStr=m.datatype.slice
  f : Outport
  wires:
  int_presc/1 -> fp_prepend_zeros/1
  fp_repr_shift_prescale/1 -> Add/1
  Add/1 -> f/1, Unit Delay/1
  fp_prepend_zeros/1 -> fp_repr_shift_prescale/1
  Unit Delay/1 -> Add/2
  fdot/1 -> Unit Delay1/1, Add1/1
  half/1 -> int_presc/1
  Add1/1 -> half/1
  Unit Delay1/1 -> Add1/2

== system MHILSimTDFixpoint/slice_0/u_nlf ==
  x : Inport
  Add : Sum  OutDataTypeStr=uint64
  Add1 : Sum  OutDataTypeStr=m.datatype.slice
  Add2 : Sum  Inputs=+-  OutDataTypeStr=m.datatype.slice
  Bitwise Operator : simulink/Logic and Bit Operations/Bitwise Operator  logicop=AND  UseBitMask=on  BitMask=bitxor((bitsll(1,m.datatype.slice_sz)-1), bitsll(1,m.datatype.slice_sz - m.datatype.nlf_lut_addr_sz)-1)  BitMaskRealWorld=Stored Integer
  Bitwise Operator1 : simulink/Logic and Bit Operations/Bitwise Operator  logicop=AND  UseBitMask=on  BitMask=bitsll(1,m.datatype.slice_sz - m.datatype.nlf_lut_addr_sz)-1  BitMaskRealWorld=Stored Integer
  Bitwise Operator2 : simulink/Logic and Bit Operations/Bitwise Operator  logicop=AND  UseBitMask=on  BitMask=bitsll(1,m.datatype.nlf_lut_addr_sz)-1  BitMaskRealWorld=Stored Integer
  Constant : Constant  OutDataTypeStr=uint64
  Constant1 : Constant  OutDataTypeStr=m.datatype.const
  Data Type Conversion1 : DataTypeConversion  OutDataTypeStr=int64  ConvertRealWorld=Stored Integer (SI)
  Data Type Conversion2 : DataTypeConversion  OutDataTypeStr=fixdt(0,m.datatype.slice_sz - m.datatype.nlf_lut_addr_sz,m.datatype.slice_sz - m.datatype.nlf_lut_addr_sz)  ConvertRealWorld=Stored Integer (SI)
  Data Type Conversion3 : DataTypeConversion  OutDataTypeStr=m.datatype.slice
  Direct Lookup Table (n-D) : LookupNDDirect  NumberOfTableDimensions=1  Table=m.slice0.u_nlf.lut  TableDataTypeStr=m.datatype.nlf
  Direct Lookup Table (n-D)1 : LookupNDDirect  NumberOfTableDimensions=1  Table=m.slice0.u_nlf.lut  TableDataTypeStr=m.datatype.nlf
  Gain : Gain  Gain=m.slice0.u_nlf.presc  OutDataTypeStr=fixdt(1,m.datatype.slice_sz,m.datatype.slice_sz-1)
  Gain1 : Gain  Gain=1/(2^(m.datatype.slice_sz - m.datatype.nlf_lut_addr_sz))  OutDataTypeStr=uint64
  Gain2 : Gain  Gain=m.slice0.u_nlf.gain  OutDataTypeStr=m.datatype.slice
  Product : Product  OutDataTypeStr=m.datatype.slice
  Product1 : Product  OutDataTypeStr=m.datatype.slice
  f(x) : Outport
  wires:
  Direct Lookup Table (n-D)/1 -> Product/1
  Data Type Conversion2/1 -> Data Type Conversion3/1
  Product1/1 -> Add1/2
  Direct Lookup Table (n-D)1/1 -> Product1/1
  Bitwise Operator/1 -> Gain1/1
  Add2/1 -> Product/2
  Gain1/1 -> Add/1, Direct Lookup Table (n-D)/1
  Gain/1 -> Data Type Conversion1/1
  Data Type Conversion3/1 -> Product1/2, Add2/2
  Data Type Conversion1/1 -> Bitwise Operator1/1, Bitwise Operator/1
  Add1/1 -> Gain2/1
  Constant1/1 -> Add2/1
  Constant/1 -> Add/2
  Product/1 -> Add1/1
  Bitwise Operator1/1 -> Data Type Conversion2/1
  Add/1 -> Bitwise Operator2/1
  x/1 -> Gain/1
  Gain2/1 -> f(x)/1
  Bitwise Operator2/1 -> Direct Lookup Table (n-D)1/1

== system MHILSimTDFixpoint/slice_0/x_nlf ==
  x : Inport
  Add : Sum  OutDataTypeStr=uint64
  Add1 : Sum  OutDataTypeStr=m.datatype.slice
  Add2 : Sum  Inputs=+-  OutDataTypeStr=m.datatype.slice
  Bitwise Operator : simulink/Logic and Bit Operations/Bitwise Operator  logicop=AND  UseBitMask=on  BitMask=bitxor((bitsll(1,m.datatype.slice_sz)-1), bitsll(1,m.datatype.slice_sz - m.datatype.nlf_lut_addr_sz)-1)  BitMaskRealWorld=Stored Integer
  Bitwise Operator1 : simulink/Logic and Bit Operations/Bitwise Operator  logicop=AND  UseBitMask=on  BitMask=bitsll(1,m.datatype.slice_sz - m.datatype.nlf_lut_addr_sz)-1  BitMaskRealWorld=Stored Integer
  Bitwise Operator2 : simulink/Logic and Bit Operations/Bitwise Operator  logicop=AND  UseBitMask=on  BitMask=bitsll(1,m.datatype.nlf_lut_addr_sz)-1  BitMaskRealWorld=Stored Integer
  Constant : Constant  OutDataTypeStr=uint64
  Constant1 : Constant  OutDataTypeStr=m.datatype.const
  Data Type Conversion1 : DataTypeConversion  OutDataTypeStr=int64  ConvertRealWorld=Stored Integer (SI)
  Data Type Conversion2 : DataTypeConversion  OutDataTypeStr=fixdt(0,m.datatype.slice_sz - m.datatype.nlf_lut_addr_sz,m.datatype.slice_sz - m.datatype.nlf_lut_addr_sz)  ConvertRealWorld=Stored Integer (SI)
  Data Type Conversion3 : DataTypeConversion  OutDataTypeStr=m.datatype.slice
  Direct Lookup Table (n-D) : LookupNDDirect  NumberOfTableDimensions=1  Table=m.slice0.x_nlf.lut  TableDataTypeStr=m.datatype.nlf
  Direct Lookup Table (n-D)1 : LookupNDDirect  NumberOfTableDimensions=1  Table=m.slice0.x_nlf.lut  TableDataTypeStr=m.datatype.nlf
  Gain : Gain  Gain=m.slice0.x_nlf.presc  OutDataTypeStr=fixdt(1,m.datatype.slice_sz,m.datatype.slice_sz-1)
  Gain1 : Gain  Gain=1/(2^(m.datatype.slice_sz - m.datatype.nlf_lut_addr_sz))  OutDataTypeStr=uint64
  Gain2 : Gain  Gain=m.slice0.x_nlf.gain  OutDataTypeStr=m.datatype.slice
  Product : Product  OutDataTypeStr=m.datatype.slice
  Product1 : Product  OutDataTypeStr=m.datatype.slice
  f(x) : Outport
  wires:
  Direct Lookup Table (n-D)/1 -> Product/1
  Data Type Conversion2/1 -> Data Type Conversion3/1
  Product1/1 -> Add1/2
  Direct Lookup Table (n-D)1/1 -> Product1/1
  Bitwise Operator/1 -> Gain1/1
  Add2/1 -> Product/2
  Gain1/1 -> Add/1, Direct Lookup Table (n-D)/1
  Gain/1 -> Data Type Conversion1/1
  Data Type Conversion3/1 -> Product1/2, Add2/2
  Data Type Conversion1/1 -> Bitwise Operator1/1, Bitwise Operator/1
  Add1/1 -> Gain2/1
  Constant1/1 -> Add2/1
  Constant/1 -> Add/2
  Product/1 -> Add1/1
  Bitwise Operator1/1 -> Data Type Conversion2/1
  Add/1 -> Bitwise Operator2/1
  x/1 -> Gain/1
  Gain2/1 -> f(x)/1
  Bitwise Operator2/1 -> Direct Lookup Table (n-D)1/1

== system MHILSimTDFixpoint/slice_0/xdot_nlf ==
  x : Inport
  Add : Sum  OutDataTypeStr=uint64
  Add1 : Sum  OutDataTypeStr=m.datatype.slice
  Add2 : Sum  Inputs=+-  OutDataTypeStr=m.datatype.slice
  Bitwise Operator : simulink/Logic and Bit Operations/Bitwise Operator  logicop=AND  UseBitMask=on  BitMask=bitxor((bitsll(1,m.datatype.slice_sz)-1), bitsll(1,m.datatype.slice_sz - m.datatype.nlf_lut_addr_sz)-1)  BitMaskRealWorld=Stored Integer
  Bitwise Operator1 : simulink/Logic and Bit Operations/Bitwise Operator  logicop=AND  UseBitMask=on  BitMask=bitsll(1,m.datatype.slice_sz - m.datatype.nlf_lut_addr_sz)-1  BitMaskRealWorld=Stored Integer
  Bitwise Operator2 : simulink/Logic and Bit Operations/Bitwise Operator  logicop=AND  UseBitMask=on  BitMask=bitsll(1,m.datatype.nlf_lut_addr_sz)-1  BitMaskRealWorld=Stored Integer
  Constant : Constant  OutDataTypeStr=uint64
  Constant1 : Constant  OutDataTypeStr=m.datatype.const
  Data Type Conversion1 : DataTypeConversion  OutDataTypeStr=int64  ConvertRealWorld=Stored Integer (SI)
  Data Type Conversion2 : DataTypeConversion  OutDataTypeStr=fixdt(0,m.datatype.slice_sz - m.datatype.nlf_lut_addr_sz,m.datatype.slice_sz - m.datatype.nlf_lut_addr_sz)  ConvertRealWorld=Stored Integer (SI)
  Data Type Conversion3 : DataTypeConversion  OutDataTypeStr=m.datatype.slice
  Direct Lookup Table (n-D) : LookupNDDirect  NumberOfTableDimensions=1  Table=m.slice0.xd_nlf.lut  TableDataTypeStr=m.datatype.nlf
  Direct Lookup Table (n-D)1 : LookupNDDirect  NumberOfTableDimensions=1  Table=m.slice0.xd_nlf.lut  TableDataTypeStr=m.datatype.nlf
  Gain : Gain  Gain=m.slice0.xd_nlf.presc  OutDataTypeStr=fixdt(1,m.datatype.slice_sz,m.datatype.slice_sz-1)
  Gain1 : Gain  Gain=1/(2^(m.datatype.slice_sz - m.datatype.nlf_lut_addr_sz))  OutDataTypeStr=uint64
  Gain2 : Gain  Gain=m.slice0.xd_nlf.gain  OutDataTypeStr=m.datatype.slice
  Product : Product  OutDataTypeStr=m.datatype.slice
  Product1 : Product  OutDataTypeStr=m.datatype.slice
  f(x) : Outport
  wires:
  Direct Lookup Table (n-D)/1 -> Product/1
  Data Type Conversion2/1 -> Data Type Conversion3/1
  Product1/1 -> Add1/2
  Direct Lookup Table (n-D)1/1 -> Product1/1
  Bitwise Operator/1 -> Gain1/1
  Add2/1 -> Product/2
  Gain1/1 -> Add/1, Direct Lookup Table (n-D)/1
  Gain/1 -> Data Type Conversion1/1
  Data Type Conversion3/1 -> Product1/2, Add2/2
  Data Type Conversion1/1 -> Bitwise Operator1/1, Bitwise Operator/1
  Add1/1 -> Gain2/1
  Constant1/1 -> Add2/1
  Constant/1 -> Add/2
  Product/1 -> Add1/1
  Bitwise Operator1/1 -> Data Type Conversion2/1
  Add/1 -> Bitwise Operator2/1
  x/1 -> Gain/1
  Gain2/1 -> f(x)/1
  Bitwise Operator2/1 -> Direct Lookup Table (n-D)1/1

== system MHILSimTDFixpoint/slice_0/xdot_presc ==
  in : Inport
  cast_to_fp_slice : DataTypeConversion  OutDataTypeStr=m.datatype.slice
  mul_presc : Gain  Gain=m.slice0.xd_presc_mul  OutDataTypeStr=m.datatype.slice
  shift_presc : Gain  Gain=2^(-m.slice0.xd_presc_bitshift)  ParamDataTypeStr=uint64  OutDataTypeStr=m.datatype.accum
  out : Outport
  wires:
  in/1 -> shift_presc/1
  cast_to_fp_slice/1 -> mul_presc/1
  shift_presc/1 -> cast_to_fp_slice/1
  mul_presc/1 -> out/1

== system MHILSimTDFixpoint/slice_0/xdot_presc1 ==
  in : Inport
  cast_to_fp_slice : DataTypeConversion  OutDataTypeStr=m.datatype.slice
  mul_presc : Gain  Gain=m.slice0.x_presc_mul  OutDataTypeStr=m.datatype.slice
  shift_presc : Gain  Gain=2^(-m.slice0.x_presc_bitshift)  ParamDataTypeStr=uint64  OutDataTypeStr=m.datatype.accum
  out : Outport
  wires:
  in/1 -> shift_presc/1
  cast_to_fp_slice/1 -> mul_presc/1
  shift_presc/1 -> cast_to_fp_slice/1
  mul_presc/1 -> out/1

== system MHILSimTDFixpoint/slice_1/int_xddot_xdot ==
  fdot : Inport
  Add : Sum  OutDataTypeStr=m.datatype.accum
  Add1 : Sum  Inputs=+-  OutDataTypeStr=m.datatype.slice
  Add2 : Sum  OutDataTypeStr=m.datatype.slice
  Unit Delay : UnitDelay  SampleTime=m.t_s  HasFrameUpgradeWarning=on
  Unit Delay1 : UnitDelay  SampleTime=m.t_s  HasFrameUpgradeWarning=on
  fp_prepend_zeros : DataTypeConversion  OutDataTypeStr=fixdt(1,m.datatype.slice_sz+m.int_scale_bits,m.datatype.slice_bin)
  fp_repr_shift_prescale : Gain  Gain=1/(2^m.int_scale_bits)  OutDataTypeStr=m.datatype.accum
  half : Gain  Gain=1/2  OutDataTypeStr=m.datatype.slice
  int_presc : Gain  Gain=m.int_dt_residual  OutDataTypeStr=m.datatype.slice
  f : Outport
  wires:
  int_presc/1 -> fp_prepend_zeros/1
  fp_repr_shift_prescale/1 -> Add/1
  Add/1 -> f/1, Unit Delay/1
  fp_prepend_zeros/1 -> fp_repr_shift_prescale/1
  Unit Delay/1 -> Add/2
  fdot/1 -> half/1, Add2/1
  Add1/1 -> int_presc/1
  Add2/1 -> Add1/1
  half/1 -> Add2/2, Unit Delay1/1
  Unit Delay1/1 -> Add1/2

== system MHILSimTDFixpoint/slice_1/int_xdot_x ==
  fdot : Inport
  Add : Sum  OutDataTypeStr=m.datatype.accum
  Add1 : Sum  OutDataTypeStr=m.datatype.slice
  Unit Delay : UnitDelay  SampleTime=m.t_s  HasFrameUpgradeWarning=on
  Unit Delay1 : UnitDelay  SampleTime=m.t_s  HasFrameUpgradeWarning=on
  fp_prepend_zeros : DataTypeConversion  OutDataTypeStr=fixdt(1,m.datatype.slice_sz+m.int_scale_bits,m.datatype.slice_bin)
  fp_repr_shift_prescale : Gain  Gain=1/(2^m.int_scale_bits)  OutDataTypeStr=m.datatype.accum
  half : Gain  Gain=1/2  OutDataTypeStr=m.datatype.slice
  int_presc : Gain  Gain=m.int_dt_residual  OutDataTypeStr=m.datatype.slice
  f : Outport
  wires:
  int_presc/1 -> fp_prepend_zeros/1
  fp_repr_shift_prescale/1 -> Add/1
  Add/1 -> f/1, Unit Delay/1
  fp_prepend_zeros/1 -> fp_repr_shift_prescale/1
  Unit Delay/1 -> Add/2
  fdot/1 -> Unit Delay1/1, Add1/1
  half/1 -> int_presc/1
  Add1/1 -> half/1
  Unit Delay1/1 -> Add1/2
